simulink model "example_House_Simple"  (R2013b)
settings: Solver=ode45  StartTime=0.0  StopTime=5*24*3600  MaxStep=600  RelTol=1e-4  AbsTol=1e-6
libraries: carnot x4
settings Model: Creator=drhf  LastModifiedBy=drhf
settings SolverCC: ZeroCrossAlgorithm=Adaptive
settings OptimizationCC: ExpressionDepthLimit=2147483647
settings DebuggingCC: StateNameClashWarn=warning
settings GRTTargetCC: CombineOutputUpdateFcns=off  GRTInterface=on

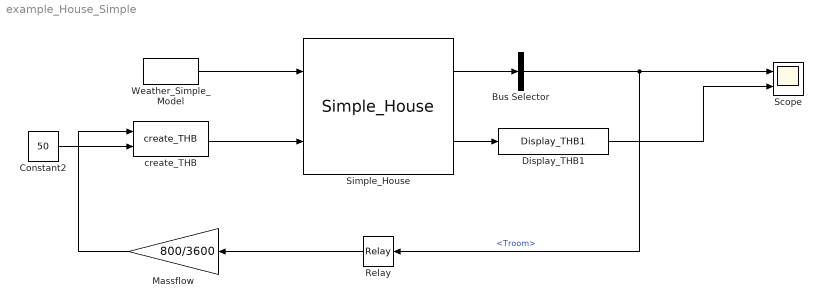
== system example_House_Simple ==
  Bus Selector : BusSelector  OutputSignals=Troom
  Constant2 : Constant  Value=50
  Display_THB1 : carnot/Outputs/Display_THB1  t=off  m=on  p=off  id=off  mix=off  d=off
  Massflow : Gain  Gain=800/3600
  Relay : Relay  OnSwitchValue=20.2  OffSwitchValue=19.8  OnOutputValue=0  OffOutputValue=1
  Scope : Scope  NumInputPorts=2
      settings: YMin=22.6~-5  YMax=24.1~5
  Simple_House : carnot/Load/Houses/Simple_House  Ahabit=140  Hroom=2.6  Floorsize=[7 10]  UAwall=0.162*(54.6+26.4)+0.182*((45.7+56.0)*2 -(12+4+3+4))  UAneighbour=0  Uground=0.18  mc=0.5e6*140 % 0.5 MJ/m2/K  shade=0.75  tini=20  Awin=[12 4 3 4]  AziWin=[0 90 -180 -90]  Uwin="[1    1   1    1]*1.0"  Gwin="[1    1   1    1]*0.585*(1-0.15)"  vent=0.4  rec=0.6  heatload=1792  dpcoeff=[10 100]  delta_t_nom=15  n_rad=1.1  mass_times_cap=40e6
  Weather_Simple_Model : carnot/Weather/Weather_Simple_Model  lat=60  Ibn=900  Idg=100  tamb=5  deltaTsky=-6  rh=50  precip="10e-3/24/3600           % 10 mm in 24 h"  cloud=0.125  p=1013e2  vw=1  wdir=270
  create_THB : carnot/Source/Simple/create_THB  p=1e5  fluid=Water  mix=0  dia=0.02  mID=No Pressure Drop
  wires:
  Bus Selector/1 -> Relay/1, Scope/1  "<Troom>"
  Constant2/1 -> create_THB/2
  Weather_Simple_Model/1 -> Simple_House/1
  create_THB/1 -> Simple_House/2
  Simple_House/1 -> Bus Selector/1
  Simple_House/2 -> Display_THB1/1
  Massflow/1 -> create_THB/1
  Relay/1 -> Massflow/1
  Display_THB1/1 -> Scope/2
